simulink library "sf_gui_elevator_controller_lib"  (Simulink 7.6)
settings: Solver=FixedStepDiscrete  StartTime=0.0  StopTime=10.0  FixedStep=1  RelTol=1e-3
undefined symbols (not defined in the file or in its folder): carID
settings Model: Creator=The MathWorks Inc.

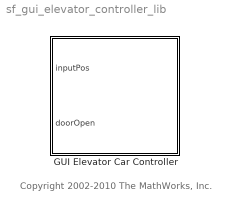
== system sf_gui_elevator_controller_lib ==
  note: Copyright 2002-2010 The MathWorks, Inc.
  GUI Elevator Car Controller : Stateflow chart  TreatAsAtomicUnit=on  mask(Stateflow){carID=carID}
      mask prompts: carID "Value for 'carID'"
      mask help: Stateflow diagram

== stateflow chart GUI Elevator Car Controller ==
  state Controller
    state move(pos) [function]
      (default) -> (junction 24) : {ml.sf_elevator_gui('move_car', carID, pos);}
    state open_door [function]
      (default) -> (junction 22) : {ml.sf_elevator_gui('open_door', carID);}
    state close_door [function]
      (default) -> (junction 23) : {ml.sf_elevator_gui('close_door', carID);}
    state deactivate_hall_button(pos) [function]
      (default) -> (junction 25) : {ml.sf_elevator_gui('deactivate', 'hall', get_floor_number(pos));}
    state deactivate_car_button(pos) [function]
      (default) -> (junction 26) : {floorNum = get_floor_number(pos);
          | ml.sf_elevator_gui('deactivate',carID, floorNum);}
    state floorNumber = get_floor_number(pos) [function]
      (default) -> (junction 27) : {floorNumber = ml.round(pos);}
    (junction 10) -> (junction 11) [order 1] : [hasChanged(inputPos)]
    (junction 10) -> (junction 12) [order 2]
    (junction 11) -> (junction 13) : {move(inputPos);}
    (junction 13) -> (junction 12)
    (junction 12) -> (junction 14)
    (junction 14) -> (junction 15) [order 1] : [hasChanged(doorOpen)]
    (junction 15) -> (junction 16)
    (junction 16) -> (junction 17) [order 1] : [doorOpen]
    (junction 16) -> (junction 19) [order 2] : {close_door();}
    (junction 17) -> (junction 20) : {open_door();}
    (junction 19) -> (junction 18) : {deactivate_hall_button(inputPos);
        |  deactivate_car_button(inputPos);}
    (junction 20) -> (junction 19)
    Controller -> (junction 10)
    (junction 14) -> (junction 18) [order 2]
    (junction 18) -> (junction 21)
  data: pos function_input double; pos function_input double; pos function_input double; floorNum temporary double; pos function_input double; floorNumber function_output double; inputPos input double; doorOpen input double; carID parameter double
